simulink model "EjemploServidorConPioneerM2011b"  (Simulink 7.8)
settings: Solver=ode3  StartTime=0.0  StopTime=inf  FixedStep=0.001  RelTol=1e-3
libraries: aerolibanimutils x1
settings Model: Creator=Usuario  LastModifiedBy=Sebastián
settings OptimizationCC: SimCompilerOptimization=On
settings CodeAppCC: CustomSymbolStrType=$N$R$M_T

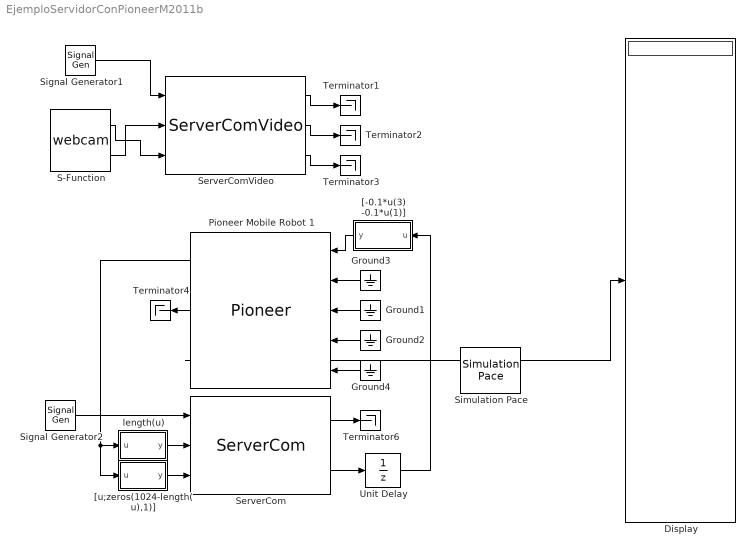
== system EjemploServidorConPioneerM2011b ==
  Display : Display
  Ground{1..4} (4 alike) : Ground
  Pioneer Mobile Robot 1 : S-Function  FunctionName=Pioneer  Parameters=1  EnableBusSupport=off
      mask Display:
      | color('red')
      | port_label('input',1,'acciones')
      | port_label('input',2,'postura')
      | port_label('input',3,'parametros')
      | port_label('input',4,'parametrosSend')
      | port_label('input',5,'posturaSend')
      | color('blue')
      | port_label('output',1,'estado')
      | port_label('output',2,'parametros')
      | port_label('output',3,'laser')
  S-Function : S-Function  FunctionName=webcam  Parameters=1  EnableBusSupport=off
  ServerCom : S-Function  FunctionName=ServerCom  EnableBusSupport=off
      mask Display:
      | patch([0 4. 4 0],[0.02 0.02 0.98 0.98],0.9*[123 193 255]/255)
      | patch([0 4 4 0],[0.1 0.1 0.9 0.9],[123 193 255]/255)
      | patch([1.5 2.5 2.5 2.3 2.3 1.7 1.7 1.5],[0 0 1 1 1.2 1.2 1 1],[130 130 130]/255)
      | patch([1.3 2.7 2.7 1.3],[1.2 1.2 2.9 2.9],0.85*[130 130 130]/255)
      | patch([1.4 2.6 2.6 1.4],[1.3 1.3 2.8 2.8],[123 193 255]/255)
      | patch([1.5 2.5 2.5 1.5],[1.4 1.4 2.7 2.7],0.85*[130 130 130]/255)
      | patch([1.9 2.1 2.1 1.9],[1.8 1.8 2.1 2.1],[123 193 255]/255)
      | color('red')
      | port_label('input',1,'clock')
      | port_label('input',2,'sizeSend')
      | port_label('input',3,'dataSend')
      | port_label('output',1,'stateChannel')
      | port_label('output',2,'dataRecv')
  ServerComVideo : S-Function  FunctionName=ServerComVideo  EnableBusSupport=off
      mask Display:
      | patch([0 4. 4 0],[0.02 0.02 0.98 0.98],0.9*[123 193 255]/255)
      | patch([0 4 4 0],[0.1 0.1 0.9 0.9],[123 193 255]/255)
      | patch([1.5 2.5 2.5 2.3 2.3 1.7 1.7 1.5],[0 0 1 1 1.2 1.2 1 1],[130 130 130]/255)
      | patch([1.3 2.7 2.7 1.3],[1.2 1.2 2.9 2.9],0.85*[130 130 130]/255)
      | patch([1.4 2.6 2.6 1.4],[1.3 1.3 2.8 2.8],[123 193 255]/255)
      | patch([1.5 2.5 2.5 1.5],[1.4 1.4 2.7 2.7],0.85*[130 130 130]/255)
      | patch([1.9 2.1 2.1 1.9],[1.8 1.8 2.1 2.1],[123 193 255]/255)
      | color('red')
      | port_label('input',1,'clock')
      | port_label('input',2,'sizeSend')
      | port_label('input',3,'dataSend')
      | port_label('output',1,'stateChannel')
      | port_label('output',2,'sizeMustBeRecv')
      | port_label('output',3,'dataRecv')
  Signal Generator1 : SignalGenerator  WaveForm=square  Frequency=20
  Signal Generator2 : SignalGenerator  WaveForm=square  Frequency=20
  Simulation Pace : aerolibanimutils/Simulation Pace  SimulationPace=1  SleepMode=MATLAB Thread  OutputPaceError=off  SampleTime=-1
      settings: AttributesFormatString=%<SimulationPace> sec/sec
  Terminator{1..4,6} (5 alike) : Terminator
  Unit Delay : UnitDelay  SampleTime=-1
  "[-0.1*u(3) -0.1*u(1)]" : MATLAB Function  TreatAsAtomicUnit=on
  "[u;zeros(1024-length(u),1)]" : MATLAB Function  TreatAsAtomicUnit=on
  length(u) : MATLAB Function  TreatAsAtomicUnit=on
  wires:
  Signal Generator1/1 -> ServerComVideo/1
  S-Function/2 -> ServerComVideo/2
  S-Function/1 -> ServerComVideo/3
  ServerComVideo/1 -> Terminator1/1
  ServerComVideo/2 -> Terminator2/1
  ServerComVideo/3 -> Terminator3/1
  "[u;zeros(1024-length(u),1)]"/1(y) -> ServerCom/3
  Pioneer Mobile Robot 1/1 -> "[u;zeros(1024-length(u),1)]"/1(u), length(u)/1(u)
  Signal Generator2/1 -> ServerCom/1
  length(u)/1(y) -> ServerCom/2
  Pioneer Mobile Robot 1/2 -> Terminator4/1
  Pioneer Mobile Robot 1/3 -> Display/1
  Ground3/1 -> Pioneer Mobile Robot 1/2
  Ground1/1 -> Pioneer Mobile Robot 1/3
  Ground2/1 -> Pioneer Mobile Robot 1/4
  Ground4/1 -> Pioneer Mobile Robot 1/5
  "[-0.1*u(3) -0.1*u(1)]"/1(y) -> Pioneer Mobile Robot 1/1
  ServerCom/2 -> Unit Delay/1
  ServerCom/1 -> Terminator6/1
  Unit Delay/1 -> "[-0.1*u(3) -0.1*u(1)]"/1(u)

== matlab function length(u) ==
  data: u input double; y output double
function y = fcn(u)
%#codegen

y = uint32(length(u));

== matlab function [u;zeros(1024-length(u),1)] ==
  data: u input double; y output double
function y = fcn(u)
%#codegen

y = [u;zeros(1024-length(u),1)];

== matlab function [-0.1*u(3) -0.1*u(1)] ==
  data: u input double; y output double
function y = fcn(u)
%#codegen

y = [u(3);u(1)];
